simulink model "Es1_sim"  (R2024a)
settings: Solver=VariableStepAuto  StartTime=0  StopTime=3400  FixedStep=1  MaxStep=0.001  RelTol=0.001
values from neighbouring files (symbols this model uses):
  scelta = menu("Scegli che caso analizzare:",'A: C=c e D=0', 'B: C=0 e D=d', 'C: C=c/x e D=0', 'D: C=0 e D=d/y', 'E: C=0 e D=0')    [Es1.m]
  val_iniziali = [5,5]    [Es1.m]
settings Model: PacingRate=1000  Creator=ferra  LastModifiedBy=eldemaster
settings HardwareCC: ProdBitPerLong=64  ProdHWDeviceType=Apple->ARM64
settings RTWCC: GPUComputeCapability=3.5

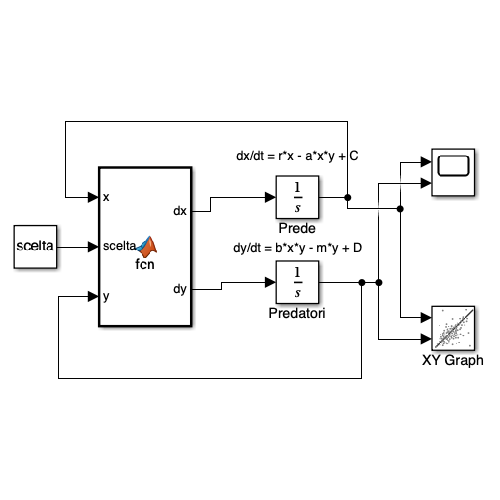
[thumbnail: Simulink's stored preview of the top-level diagram]
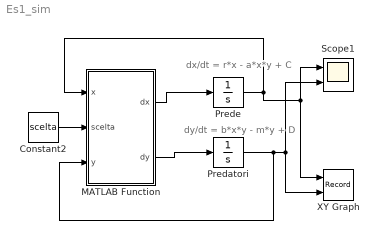
== system Es1_sim ==
  note: dx/dt = r*x - a*x*y + C
  note: dy/dt = b*x*y - m*y + D
  Constant2 : Constant  Value=scelta
  MATLAB Function : MATLAB Function  TreatAsAtomicUnit=on
  Predatori : Integrator  InitialCondition=val_iniziali(1)  UpperSaturationLimit=34
  Prede : Integrator  InitialCondition=val_iniziali(1)  UpperSaturationLimit=34
  Scope1 : Scope  NumInputPorts=2
  XY Graph : Record  FileSettingsInternal="{\"entries\":[{\"content\":{\"excelSettings\":{\"content\":{},\"type\":\"Streamout.ExcelSettings\"}},\"type\":\"Streamout.FileSettingStorage\",\"uuid\":\"\"}],\"packageUris\":[\"http:\\/\\/schema.mathworks.com\\/mf0\\/streamout_blocks\\/R2020a\"],\"version\":\"1.0\"}"  Layout=[1 1]  SignalsInternal="{\"entries\":[{\"content\":{\"signals\":[{\"content\":{\"blockPath\":[],\"dimensions\":[1],\"domain\":\"\",\"lineColor\":\"#a2142f\",\"plots\":[ 1 ],\"port\":1,\"sid\":[\"\"],\"signalID\":1,\"signalName\":\"Prede\"},\"type\":\"RecordBlkView.Signal\",\"uuid\":\"\"},{\"content\":{\"blockPath\":[],\"dimensions\":[1],\"domain\":\"\",\"lineColor\":\"#139fff\",\"plots\":[ 1 ],\"port\":2,\"sid\":[\"\"],\"signalID\":2,\"signalName\":\"Predatori\"},\"type\":\"RecordBlkView.Signal\",\"uuid\":\"\"}]},\"type\":\"RecordBlkView.InputSignals\",\"uuid\":\"\"}],\"packageUris\":[\"http:\\/\\/schema.mathworks.com\\/mf0\\/streamout_blocks\\/R2020a\"],\"version\":\"1.0\"}"  VisualizationBindings="{\"xyplotplugin\":{\"info\":[{\"series\":[{\"bindingParametersList\":[{\"parameter\":\"X-Axis\",\"signalID\":1,\"signalName\":\"Prede\"},{\"parameter\":\"Y-Axis\",\"signalID\":2,\"signalName\":\"Predatori\"}],\"seriesID\":0}],\"subplotID\":1}]}}"  CompatibilityTag=XY  st=-1
  wires:
  MATLAB Function/1(dx) -> Prede/1
  Prede/1 -> XY Graph/1, Scope1/1, MATLAB Function/1(x)
  Constant2/1 -> MATLAB Function/2(scelta)
  Predatori/1 -> MATLAB Function/3(y), Scope1/2, XY Graph/2
  MATLAB Function/2(dy) -> Predatori/1

== matlab function Es1_sim/MATLAB Function ==
  data: x input; scelta input; y input; dx output; dy output
function [dx, dy]= fcn(x, scelta, y)

dx = 0;
dy = 0;
r = 0.1; 
a = 0.1; 
b = 0.3; 
m = 0.2;

c = 0.01;
d= 0.01;


switch scelta

      case 1 %CASO A

          C = c;
          D = 0;

          dx = r*x - a*x*y + C;
          dy = b*x*y - m*y + D;

        

      case 2 %CASO B

          C = 0;
          D = d;

          dx = r*x - a*x*y + C;
          dy = b*x*y - m*y + D;


     

      case 3 %CASO C

          C = c/x;
          D = 0;

          dx = r*x - a*x*y + C;
          dy = b*x*y - m*y + D;

    

      case 4 %CASO D

          C = 0;
          D = d/y;
          
          dx = r*x - a*x*y + C;
          dy = b*x*y - m*y + D;
     
      case 5  %CASO E

          C = 0;
          D = 0;
          dx = r*x - a*x*y;
          dy = b*x*y - m*y;


end
